simulink model "V2_Pneumatikzylinder_Sim_Template"  (R2024a)
settings: Solver=FixedStepAuto  StartTime=0.0  StopTime=3  FixedStep=1e-3  RelTol=1e-3
values from neighbouring files (symbols this model uses):
  A = pi*d^2/4    (= 0.00125663706144)    [Hilfsskript.m]    (also in V2_Pneumatikzylinder_ini_Template.m)
  a0s = double(solution.a0)    [V2_Pneumatikzylinder_ini_Template.m]
  a1s = double(solution.a1)    [V2_Pneumatikzylinder_ini_Template.m]
  a2s = double(solution.a2)    [V2_Pneumatikzylinder_ini_Template.m]
  a3s = double(solution.a3)    [V2_Pneumatikzylinder_ini_Template.m]
  a4s = double(solution.a4)    [V2_Pneumatikzylinder_ini_Template.m]
  a5s = double(solution.a5)    [V2_Pneumatikzylinder_ini_Template.m]
  b_0 = 50    [Hilfsskript.m]    (also in V2_Pneumatikzylinder_ini_Template.m)
  b_1 = 20    [Hilfsskript.m]    (also in V2_Pneumatikzylinder_ini_Template.m)
  F_C = 10    [Hilfsskript.m]    (also in V2_Pneumatikzylinder_ini_Template.m)
  F_S = 5    [Hilfsskript.m]    (also in V2_Pneumatikzylinder_ini_Template.m)
  gamma_1 = 300    [V2_Pneumatikzylinder_ini_Template.m]
  gamma_2 = 200    [V2_Pneumatikzylinder_ini_Template.m]
  gamma_3 = 2000    [V2_Pneumatikzylinder_ini_Template.m]
  gamma_p = 500    [V2_Pneumatikzylinder_ini_Template.m]
  L = 0.5    [Hilfsskript.m]    (also in V2_Pneumatikzylinder_ini_Template.m)
  m = 1.7    [Hilfsskript.m]    (also in V2_Pneumatikzylinder_ini_Template.m)
  n = 1    [Hilfsskript.m]    (also in V2_Pneumatikzylinder_ini_Template.m)
  p0 = 1e5    (= 100000)    [Hilfsskript.m]    (also in V2_Pneumatikzylinder_ini_Template.m)
  pm = 3.5e5    (= 350000)    [Hilfsskript.m]    (also in V2_Pneumatikzylinder_ini_Template.m)
  R = 287.058    [Hilfsskript.m]    (also in V2_Pneumatikzylinder_ini_Template.m)
  S_gain = 1 / dcgain(sys_disc_cont)    [V2_Pneumatikzylinder_ini_Template.m]
  T0 = 293.15    [Hilfsskript.m]    (also in V2_Pneumatikzylinder_ini_Template.m)
  u_sim = SISO_MOLE.u_cell{idx_u}    [V2_Pneumatikzylinder_ini_Template.m]
  V0 = 1e-5    (= 1e-05)    [Hilfsskript.m]    (also in V2_Pneumatikzylinder_ini_Template.m)
  v_S = 1e-3    (= 0.001)    [Hilfsskript.m]    (also in V2_Pneumatikzylinder_ini_Template.m)
undefined symbols (not defined in the file or in its folder): ref_traj
settings Model: Creator=Alexander Wache  LastModifiedBy=oleup
settings SolverCC: AlgebraicLoopSolver=TrustRegion
settings DataIOCC: ReturnWorkspaceOutputs=off
settings OptimizationCC: ReuseModelBlockBuffer=off
settings DebuggingCC: UnconnectedInputMsg=warning  UnconnectedOutputMsg=warning  UnconnectedLineMsg=warning  ArithmeticOperatorsInVariantConditions=warning
settings ModelReferenceCC: EnableRefExpFcnMdlSchedulingChecks=on
settings SFSimCC: CustomCodeUndefinedFunction=UseInterfaceOnly
settings RTWCC: GPUComputeCapability=3.5  DLArmComputeVersion=19.05

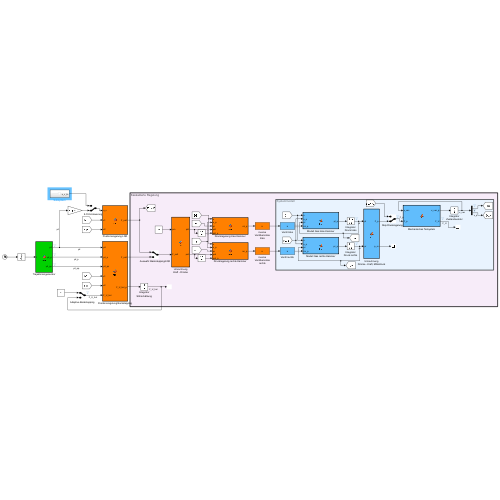
[thumbnail: Simulink's stored preview of the top-level diagram]
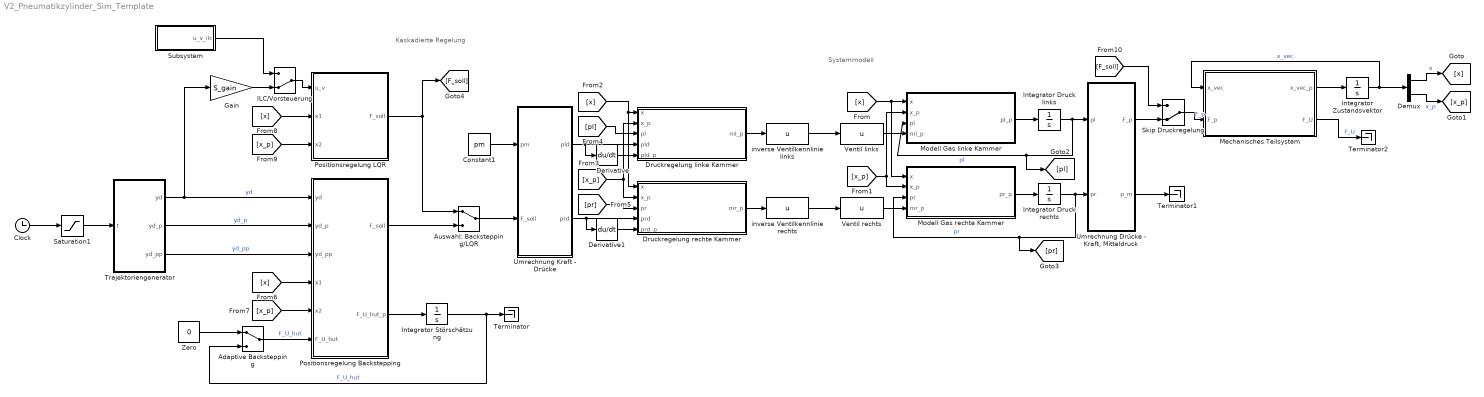
== system V2_Pneumatikzylinder_Sim_Template ==
  note: Kaskadierte Regelung
  note: Systemmodell
  Adaptive Backstepping : ManualSwitch
  Auswahl: Backstepping/LQR : ManualSwitch
  Clock : Clock
  Constant1 : Constant  Value=pm
  Demux : Demux  Outputs=2
  Derivative : Derivative
  Derivative1 : Derivative
  Druckregelung linke Kammer : MATLAB Function  TreatAsAtomicUnit=on
  Druckregelung rechte Kammer : MATLAB Function  TreatAsAtomicUnit=on
  Gain : Gain  Gain=S_gain
  ILC/Vorsteuerung : ManualSwitch  CurrentSetting=0
  Integrator Druck links : Integrator  InitialCondition=p0  LimitOutput=on  LowerSaturationLimit=1e4
  Integrator Druck rechts : Integrator  InitialCondition=p0  LimitOutput=on  LowerSaturationLimit=1e4
  Integrator Störschätzung : Integrator  LowerSaturationLimit=1e4
  Integrator Zustandsvektor : Integrator  InitialCondition=[0.1, 0]
  Mechanisches Teilsystem : MATLAB Function  TreatAsAtomicUnit=on
  Modell Gas linke Kammer : MATLAB Function  TreatAsAtomicUnit=on
  Modell Gas rechte Kammer : MATLAB Function  TreatAsAtomicUnit=on
  Positionsregelung Backstepping : MATLAB Function  TreatAsAtomicUnit=on
  Positionsregelung LQR : MATLAB Function  TreatAsAtomicUnit=on
  Saturation1 : Saturate  UpperLimit=1  LowerLimit=0
  Skip Druckregelung : ManualSwitch  CurrentSetting=0
  Subsystem : Subsystem
  Terminator : Terminator
  Terminator1 : Terminator
  Terminator2 : Terminator
  Trajektoriengenerator : MATLAB Function  TreatAsAtomicUnit=on
  "Umrechnung Drücke - Kraft, Mitteldruck" : MATLAB Function  TreatAsAtomicUnit=on
  Umrechnung Kraft - Drücke : MATLAB Function  TreatAsAtomicUnit=on
  Ventil links : Fcn  Expr=u
  Ventil rechts : Fcn  Expr=u
  Zero : Constant  Value=0  OutDataTypeStr=Inherit: Inherit via back propagation
  inverse Ventilkennlinie links : Fcn  Expr=u
  inverse Ventilkennlinie rechts : Fcn  Expr=u
  wires:
  Modell Gas linke Kammer/1(pl_p) -> Integrator Druck links/1
  Modell Gas rechte Kammer/1(pr_p) -> Integrator Druck rechts/1
  Clock/1 -> Saturation1/1
  Saturation1/1 -> Trajektoriengenerator/1(t)
  Positionsregelung Backstepping/2(F_U_hut_p) -> Integrator Störschätzung/1
  Integrator Störschätzung/1 -> Terminator/1, Adaptive Backstepping/2  "F_U_hut"
  Mechanisches Teilsystem/1(x_vec_p) -> Integrator Zustandsvektor/1
  Integrator Zustandsvektor/1 -> Demux/1, Mechanisches Teilsystem/1(x_vec)  "x_vec"
  Demux/1 -> [x]  "x"
  Demux/2 -> [x_p]  "x_p"
  inverse Ventilkennlinie links/1 -> Ventil links/1
  inverse Ventilkennlinie rechts/1 -> Ventil rechts/1
  Ventil links/1 -> Modell Gas linke Kammer/4(ml_p)
  Ventil rechts/1 -> Modell Gas rechte Kammer/4(mr_p)
  Derivative/1 -> Druckregelung linke Kammer/5(pld_p)
  Derivative1/1 -> Druckregelung rechte Kammer/5(prd_p)
  "Umrechnung Drücke - Kraft, Mitteldruck"/2(p_m) -> Terminator1/1
  [x] -> Modell Gas linke Kammer/1(x), Modell Gas rechte Kammer/1(x)
  [x_p] -> Modell Gas rechte Kammer/2(x_p), Modell Gas linke Kammer/2(x_p)
  Integrator Druck links/1 -> Modell Gas linke Kammer/3(pl), [pl], "Umrechnung Drücke - Kraft, Mitteldruck"/1(pl)  "pl"
  Integrator Druck rechts/1 -> Modell Gas rechte Kammer/3(pr), [pr], "Umrechnung Drücke - Kraft, Mitteldruck"/2(pr)  "pr"
  Druckregelung linke Kammer/1(ml_p) -> inverse Ventilkennlinie links/1
  Druckregelung rechte Kammer/1(mr_p) -> inverse Ventilkennlinie rechts/1
  Umrechnung Kraft - Drücke/1(pld) -> Derivative/1, Druckregelung linke Kammer/4(pld)
  Umrechnung Kraft - Drücke/2(prd) -> Derivative1/1, Druckregelung rechte Kammer/4(prd)
  [x] -> Druckregelung rechte Kammer/1(x), Druckregelung linke Kammer/1(x)
  [x_p] -> Druckregelung rechte Kammer/2(x_p), Druckregelung linke Kammer/2(x_p)
  [pl] -> Druckregelung linke Kammer/3(pl)
  [pr] -> Druckregelung rechte Kammer/3(pr)
  Constant1/1 -> Umrechnung Kraft - Drücke/1(pm)
  [x] -> Positionsregelung Backstepping/4(x1)
  [x_p] -> Positionsregelung Backstepping/5(x2)
  Trajektoriengenerator/1(yd) -> Positionsregelung Backstepping/1(yd), Gain/1  "yd"
  Trajektoriengenerator/2(yd_p) -> Positionsregelung Backstepping/2(yd_p)  "yd_p"
  Trajektoriengenerator/3(yd_pp) -> Positionsregelung Backstepping/3(yd_pp)  "yd_pp"
  Mechanisches Teilsystem/2(F_U) -> Terminator2/1  "F_U"
  Adaptive Backstepping/1 -> Positionsregelung Backstepping/6(F_U_hut)  "F_U_hut"
  Zero/1 -> Adaptive Backstepping/1
  Auswahl: Backstepping/LQR/1 -> Umrechnung Kraft - Drücke/2(F_soll)
  Positionsregelung Backstepping/1(F_soll) -> Auswahl: Backstepping/LQR/2
  Positionsregelung LQR/1(F_soll) -> Auswahl: Backstepping/LQR/1, [F_soll]
  [x] -> Positionsregelung LQR/2(x1)
  [x_p] -> Positionsregelung LQR/3(x2)
  Skip Druckregelung/1 -> Mechanisches Teilsystem/2(F_p)  "F_p"
  "Umrechnung Drücke - Kraft, Mitteldruck"/1(F_p) -> Skip Druckregelung/2
  [F_soll] -> Skip Druckregelung/1
  Gain/1 -> ILC/Vorsteuerung/2
  ILC/Vorsteuerung/1 -> Positionsregelung LQR/1(u_v)
  Subsystem/1(u_v_ilc) -> ILC/Vorsteuerung/1

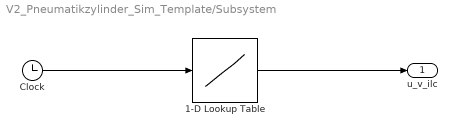
== system V2_Pneumatikzylinder_Sim_Template/Subsystem ==
  1-D Lookup Table : Lookup_n-D  NumberOfTableDimensions=1  BreakpointsForDimension1=ref_traj.t_vec  Table=u_sim  ExtrapMethod=Clip  InternalRulePriority=Speed  RndMeth=Simplest
  Clock : Clock
  u_v_ilc : Outport
  wires:
  Clock/1 -> 1-D Lookup Table/1
  1-D Lookup Table/1 -> u_v_ilc/1

== matlab function V2_Pneumatikzylinder_Sim_Template/Trajektoriengenerator ==
  data: t input; yd output; yd_p output; yd_pp output; a0s parameter; a1s parameter; a2s parameter; a3s parameter; a4s parameter; a5s parameter
function [yd, yd_p, yd_pp] = fcn(t, a0s, a1s, a2s, a3s, a4s, a5s)
% t     - Zeit

% Polynom für die Wunschposition yd
yd    = a5s*t^5 + a4s*t^4 + a3s*t^3 + a2s*t^2 + a1s*t + a0s;
% Polynom für die Wunschgeschwindigkeit yd_p
yd_p  = 5*a5s*t^4 + 4*a4s*t^3 + 3*a3s*t^2 + 2*a2s*t + a1s;
% Polynom für die Wunschbeschleunigung yd_pp
yd_pp = 20*a5s*t^3 + 12*a4s*t^2 + 6*a3s*t + 2*a2s;

== matlab function V2_Pneumatikzylinder_Sim_Template/Umrechnung Kraft - Drücke ==
  data: pm input; F_soll input; pld output; A parameter; prd output
function [pld, prd] = fcn(pm, F_soll, A)
% pm     - Pneumatischer Mitteldruck
% F_soll - Sollkraft aus äußerer Regelschleife
% A      - Kolbenfläche

% linker Solldruck für die Druckregelung
pld = pm + 1/2*F_soll/A;
% rechter Solldruck für die Druckregelung
prd = pm - 1/2*F_soll/A;

== matlab function V2_Pneumatikzylinder_Sim_Template/Positionsregelung LQR ==
  data: u_v input; F_soll output; x1 input; x2 input; k_T parameter
function F_soll  = fcn(u_v, x1, x2, k_T)
% yd    - Sollposition
% x1    - Kolbenposition (x)
% x2    - Kolbengeschwindigkeit (x_p)

% Zustandsvektor 
x = [x1;
    x2];

% Regelung
F_soll = u_v - k_T*x;

== matlab function V2_Pneumatikzylinder_Sim_Template/Umrechnung Drücke - Kraft, Mitteldruck ==
  data: pl input; F_p output; pr input; A parameter; p_m output
function [F_p, p_m] = fcn(pl, pr, A)
% pl    - linker Kammerdruck
% pr    - rechter Kammerdruck
% A     - Kolbenfläche

% Berechnung des Mitteldruckes im Zylinder (Gleichung 10)
p_m = 0.5*(pl + pr);
% Berechnung der wirkenden Zylinderkraft (Gleichung 8)
F_p = A*(pl - pr);

== matlab function V2_Pneumatikzylinder_Sim_Template/Mechanisches Teilsystem ==
  data: x_vec input; F_p input; x_vec_p output; m parameter; F_S parameter; F_C parameter; v_S parameter; b_0 parameter; b_1 parameter; F_U output
function [x_vec_p, F_U]  = fcn(x_vec, F_p, m, F_S, F_C, v_S, b_0, b_1)
% x_vec - Zustandsvektor
% F_p   - Stellgröße
% m     - Kolbenmasse
% F_S   - Stribeck-Reibung
% F_C   - Coulomb-Reibung
% v_S   - Stribeck-Geschwindigkeit
% b_0   - linearer Reibterm
% b_1   - quadratischer Reibterm

% Epsilon für Approximierung der sign() Funktion
eps = 0.01;

% Auslesen der Zustände x1 und x2 aus dem Zustandsvektor x_vec
x1 = x_vec(1);
x2 = x_vec(2);

% Berechnung des statischen Reibmodells
F_U = (F_C + (F_S - F_C)*exp(-(x2/v_S)^2))*tanh(x2/eps) + (b_0 - abs(x2)*b_1)*x2;
F_U = 0;

% Zeitableitung des ersten Zustandes
x1_p = x2;
% Zeitableitung des zweiten Zustandes
x2_p = 1/m*(F_p - F_U);

% Zusammenstellen der Zeitableitung des Zustandsvektors
x_vec_p = [x1_p; ...
           x2_p];

== matlab function V2_Pneumatikzylinder_Sim_Template/Modell Gas rechte Kammer ==
  data: pr_p output; x input; x_p input; pr input; mr_p input; n parameter; R parameter; T0 parameter; A parameter; L parameter; V0 parameter
function pr_p = fcn(x, x_p, pr, mr_p, n, R, T0, A, L, V0)
% x     - Kolbenposition
% x_p   - Kolbengeschwindigkeit
% pr    - Kammerdruck rechts
% mr_p  - Massenstrom rechts
% n     - Polytropenexponent
% R     - spefizische Gaskonstante für trockene Luft
% T0    - Gastemperatur (Umgebungstemperatur)
% A     - Kolbenfläche
% L     - Kolbenlänge
% V0    - rechtes Totvolumen

% Volumen der rechten Kammer (Gleichung 3)
Vr   = A*(L - x) + V0;
% Volumenänderung in der rechten Kammer
Vr_p = -A*x_p;
% Druckänderung in der rechten Kammer (Gleichung 4)
pr_p = n/Vr*(R*T0*mr_p - pr*Vr_p);

== matlab function V2_Pneumatikzylinder_Sim_Template/Modell Gas linke Kammer ==
  data: pl_p output; x input; x_p input; pl input; ml_p input; n parameter; R parameter; T0 parameter; A parameter; L parameter; V0 parameter
function pl_p = fcn(x, x_p, pl, ml_p, n, R, T0, A, L, V0)
% x     - Kolbenposition
% x_p   - Kolbengeschwindigkeit
% pl    - Kammerdruck links
% mlp   - Massenstrom links
% n     - Polytropenexponent
% R     - spefizische Gaskonstante für trockene Luft
% T0    - Gastemperatur (Umgebungstemperatur)
% A     - Kolbenfläche
% L     - Kolbenlänge
% V0    - linkes Totvolumen

% Volumen der linken Kammer (Gleichung 2)
Vl   = A*x + V0;
% Volumenänderung in der linken Kammer
Vl_p = A*x_p;
% Druckänderung in der linken Kammer (Gleichung 4)
pl_p = n/Vl*(R*T0*ml_p - pl*Vl_p);

== matlab function V2_Pneumatikzylinder_Sim_Template/Druckregelung linke Kammer ==
  data: ml_p output; x input; x_p input; pl input; pld input; pld_p input; n parameter; R parameter; T0 parameter; A parameter; L parameter; V0 parameter; gamma_p parameter
function ml_p = fcn(x, x_p, pl, pld, pld_p, n, R, T0, A, L, V0, gamma_p)
% x     - Kolbenposition
% x_p   - Kolbengeschwindigkeit
% pl    - Kammerdruck links
% ml_p  - Massenstrom links
% n     - Polytropenexponent
% R     - spefizische Gaskonstante für trockene Luft
% T0    - Gastemperatur (Umgebungstemperatur)
% A     - Kolbenfläche
% L     - Kolbenlänge
% V0    - linkes Totvolumen
% pld   - Soll-Druck links
% pld_p - Soll-Drückänderung links
% gamma_p   - Regelungsparameter

% linkes Kammervolumen
Vl   = A*x + V0;
% linke Kammervolumenänderung
Vl_p = A*x_p;
% Druck-Regelfehler links
e = pld - pl;
% Soll-Luftmassenstrom
ml_p = ((pld_p + gamma_p*e)*Vl/n + pl*Vl_p)*1/(R*T0);

== matlab function V2_Pneumatikzylinder_Sim_Template/Positionsregelung Backstepping ==
  data: yd input; F_soll output; yd_p input; yd_pp input; x1 input; x2 input; m parameter; gamma_1 parameter; gamma_2 parameter; F_U_hut input; F_U_hut_p output; gamma_3 parameter
function [F_soll, F_U_hut_p] = fcn(yd, yd_p, yd_pp, x1, x2, m, gamma_1, gamma_2, F_U_hut, gamma_3)
% yd    - Sollposition
% yd_p  - Sollgeschwindigkeit
% yd_pp - Sollbeschleunigung
% x1    - Kolbenposition (x)
% x2    - Kolbengeschwindigkeit (x_p)
% m     - Kolbenmasse
% gamma_1   - Reglerparameter der Positionsregelung
% gamma_2   - Reglerparameter der Geschwindigkeitsregelung
% F_U_hut   - geschätzte Störkraft
% gamma_3   - Reglerparameter der adaptiven Parameterschätzung

% Bestimmung des Ausgangsfehlers
e1   = yd - x1;
% Berechnung der virtuellen Stellgröße
x_2w = yd_p + gamma_1*e1;

% Berechnung des Fehlers in der virtuellen Stellgröße
e2     = x_2w - x2;
% Bestimmung des stabilisierenden Regelgesetzes
F_soll = m*(e1 + yd_pp + gamma_1*(-gamma_1*e1 + e2) + gamma_2*e2) + F_U_hut;

% Bestimmung der Differentialgleichung zur Schätzung des unbekannten
% Parameters F_U_p
F_U_hut_p  = 2*gamma_3*e2/m;

== matlab function V2_Pneumatikzylinder_Sim_Template/Druckregelung rechte Kammer ==
  data: mr_p output; x input; x_p input; pr input; prd input; prd_p input; n parameter; R parameter; T0 parameter; A parameter; L parameter; V0 parameter; gamma_p parameter
function mr_p = fcn(x, x_p, pr, prd, prd_p, n, R, T0, A, L, V0, gamma_p)
% x     - Kolbenposition
% x_p   - Kolbengeschwindigkeit
% pr    - Kammerdruck links
% mr_p  - Massenstrom links
% n     - Polytropenexponent
% R     - spefizische Gaskonstante für trockene Luft
% T0    - Gastemperatur (Umgebungstemperatur)
% A     - Kolbenfläche
% L     - Kolbenlänge
% V0    - linkes Totvolumen
% prd   - Soll-Druck links
% prd_p - Soll-Drückänderung links
% gamma_p   - Regelungsparameter

% rechtes Kammervolumen
Vr   = A*(L - x) + V0;
% rechte Kammervolumenänderung
Vr_p = -A*x_p;
% Druck-Regelfehler rechts
e = prd - pr;
% Soll-Luftmassenstrom
mr_p = ((prd_p + gamma_p*e)*Vr/n + pr*Vr_p)*1/(R*T0);
